simulink model "exer_2_3"  (R2014b)
settings: Solver=ode45  StartTime=0.0  StopTime=1  RelTol=1e-3
undefined symbols (not defined in the file or in its folder): get
libraries: dspspect3 x1, dspsnks4 x1
settings Model: Creator=Charlie  LastModifiedBy=Charlie

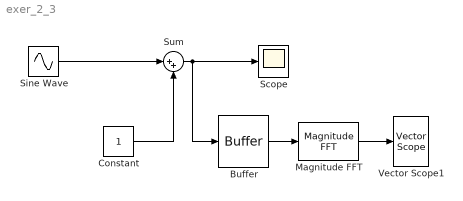
== system exer_2_3 ==
  Buffer : Buffer  N=256  TreatMby1Signals=One channel
  Constant : Constant
  Magnitude FFT : dspspect3/Magnitude FFT  mag_or_magsq=Magnitude squared  FFTImplementation=Auto  fftLenInherit=off  fftsize=256  WrapInput=on
  Scope : Scope
  Sine Wave : Sin  SineType=Sample based  Frequency=1000  Samples=302  SampleTime=1/48000
  Sum : Sum  Inputs=|++
  Vector Scope1 : dspsnks4/Vector Scope  ScopeProperties=on  Domain=Frequency  HorizSpan=1  DisplayProperties=off  AxisGrid=on  Memory=off  FrameNumber=on  AxisLegend=off  AxisZoom=off  OpenScopeAtSimStart=on  OpenScopeImmediately=off  FigPos=get(0,'defaultfigureposition')  AxisProperties=off  XUnits=Hertz  XRange=[0...Fs/2]  InheritXIncr=on  XIncr=1  XLabel=Time  XLimit=Auto  XMin=0  XMax=1  XStart=0  YUnits=dB  YLabel=Amplitude  LineProperties=off  XAxisParamsVer=6.9
      settings: YMin=-10  YMax=100
  wires:
  Constant/1 -> Sum/2
  Sine Wave/1 -> Sum/1
  Sum/1 -> Buffer/1, Scope/1
  Buffer/1 -> Magnitude FFT/1
  Magnitude FFT/1 -> Vector Scope1/1
